simulink model "pen_linear_compare"  (R2018a)
settings: Solver=VariableStepAuto  StartTime=0.0  StopTime=10.0  RelTol=1e-3
undefined symbols (not defined in the file): A, B, C, coA, coB, coC
settings Model: Creator=ros  LastModifiedBy=ros

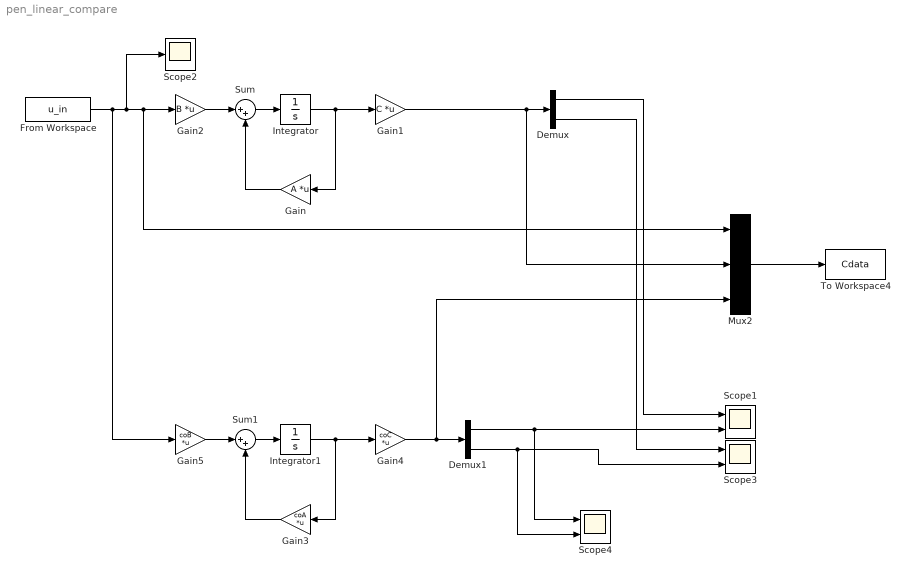
== system pen_linear_compare ==
  Demux : Demux  Outputs=2
  Demux1 : Demux  Outputs=2
  From Workspace : FromWorkspace  VariableName=u_in  SampleTime=0.001
  Gain : Gain  Gain=A  Multiplication=Matrix(K*u)
  Gain1 : Gain  Gain=C  Multiplication=Matrix(K*u)
  Gain2 : Gain  Gain=B  Multiplication=Matrix(K*u)
  Gain3 : Gain  Gain=coA  Multiplication=Matrix(K*u)
  Gain4 : Gain  Gain=coC  Multiplication=Matrix(K*u)
  Gain5 : Gain  Gain=coB  Multiplication=Matrix(K*u)
  Integrator : Integrator
  Integrator1 : Integrator
  Mux2 : Mux  Inputs=3
  Scope1 : Scope  NumInputPorts=2
  Scope2 : Scope
  Scope3 : Scope  NumInputPorts=2
  Scope4 : Scope  NumInputPorts=2
  Sum : Sum  Inputs=|++
  Sum1 : Sum  Inputs=|++
  To Workspace4 : ToWorkspace  VariableName=Cdata  SaveFormat=Timeseries  SampleTime=-1
  wires:
  Integrator/1 -> Gain1/1, Gain/1
  Gain/1 -> Sum/2
  Gain2/1 -> Sum/1
  Sum/1 -> Integrator/1
  Gain1/1 -> Mux2/2, Demux/1
  Mux2/1 -> To Workspace4/1
  Demux/1 -> Scope1/1
  Demux/2 -> Scope3/1
  Gain3/1 -> Sum1/2
  Sum1/1 -> Integrator1/1
  Integrator1/1 -> Gain4/1, Gain3/1
  Gain5/1 -> Sum1/1
  From Workspace/1 -> Gain5/1, Scope2/1, Mux2/1, Gain2/1
  Gain4/1 -> Demux1/1, Mux2/3
  Demux1/1 -> Scope4/1, Scope1/2
  Demux1/2 -> Scope4/2, Scope3/2
